simulink model "common_2"  (R2015b)
settings: Solver=ode4  StartTime=0.0  StopTime=10  FixedStep=0.005  RelTol=1e-3
undefined symbols (not defined in the file): dq_init, g, l1, l2, para, q_init
settings Model: Creator=Administrator  LastModifiedBy=Administrator

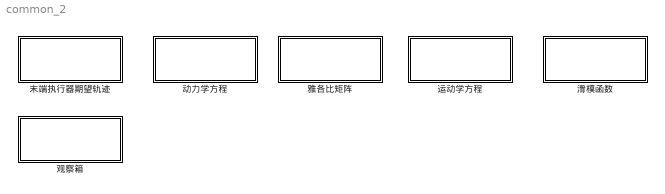
== system common_2 ==
  动力学方程 : Subsystem
      mask Display: disp('动力学方程')
  末端执行器期望轨迹 : Subsystem
      mask Display: disp('期望轨迹')
  滑模函数 : Subsystem
  观察箱 : Subsystem
  运动学方程 : Subsystem
      mask Display: disp('运动学方程')
  雅各比矩阵 : Subsystem
      mask Display: disp('雅各比矩阵')

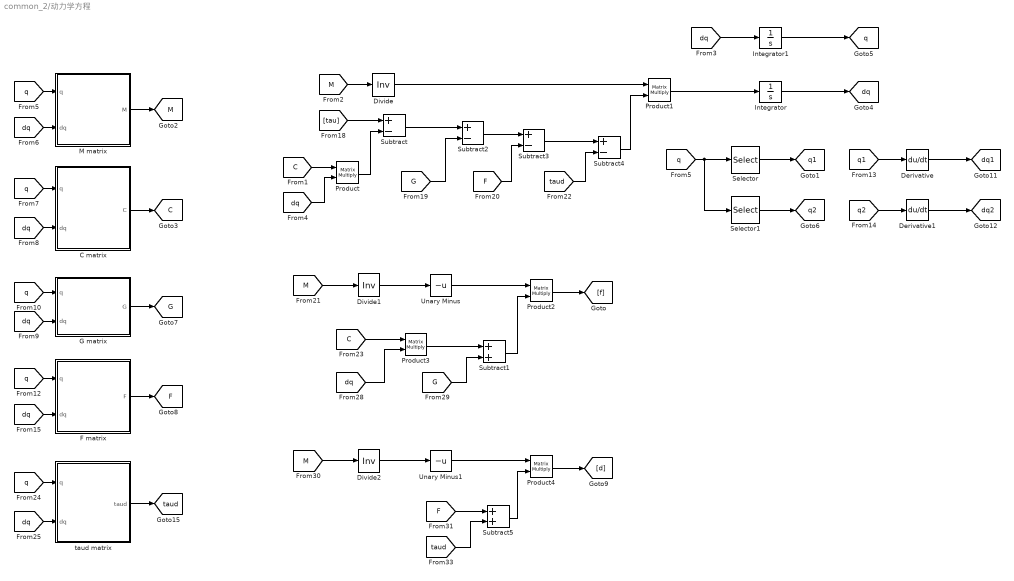
== system common_2/动力学方程 ==
  C matrix : Subsystem
  Derivative : Derivative
  Derivative1 : Derivative
  Divide : Product  Inputs=/  Multiplication=Matrix(*)
  Divide1 : Product  Inputs=/  Multiplication=Matrix(*)
  Divide2 : Product  Inputs=/  Multiplication=Matrix(*)
  F matrix : Subsystem
  G matrix : Subsystem
  Integrator : Integrator  InitialCondition=dq_init
  Integrator1 : Integrator  InitialCondition=q_init
  M matrix : Subsystem
  Product{,1..4} (5 alike) : Product  Multiplication=Matrix(*)
  Selector : Selector  InputPortWidth=2  IndexOptions=Index vector (dialog)  Indices=[1]  OutputSizes=1
  Selector1 : Selector  InputPortWidth=2  IndexOptions=Index vector (dialog)  Indices=[2]  OutputSizes=1
  Subtract{,2..4} (4 alike) : Sum  Inputs=+-
  Subtract1 : Sum
  Subtract5 : Sum
  Unary Minus : UnaryMinus
  Unary Minus1 : UnaryMinus
  taud matrix : Subsystem
  tag scope: C=global, F=global, G=global, M=global, dq1=global, dq2=global, dq=global, q1=global, q2=global, q=global, taud=global
  wires:
  Integrator/1 -> [dq]
  [dq] -> Integrator1/1
  Integrator1/1 -> [q]
  Selector/1 -> [q1]
  Selector1/1 -> [q2]
  [q] -> Selector1/1, Selector/1
  [q1] -> Derivative/1
  Derivative/1 -> [dq1]
  [q2] -> Derivative1/1
  Derivative1/1 -> [dq2]
  [q] -> C matrix/1(q)
  [dq] -> C matrix/2(dq)
  [q] -> M matrix/1(q)
  M matrix/1(M) -> [M]
  C matrix/1(C) -> [C]
  G matrix/1(G) -> [G]
  F matrix/1(F) -> [F]
  [M] -> Divide/1
  Product1/1 -> Integrator/1
  [q] -> G matrix/1(q)
  [q] -> F matrix/1(q)
  [dq] -> F matrix/2(dq)
  [q] -> taud matrix/1(q)
  [dq] -> taud matrix/2(dq)
  taud matrix/1(taud) -> [taud]
  Divide/1 -> Product1/1
  [tau] -> Subtract/1
  [C] -> Product/1
  [dq] -> Product/2
  Product/1 -> Subtract/2
  Subtract/1 -> Subtract2/1
  [G] -> Subtract2/2
  Subtract2/1 -> Subtract3/1
  [F] -> Subtract3/2
  Subtract3/1 -> Subtract4/1
  [taud] -> Subtract4/2
  Subtract4/1 -> Product1/2
  [dq] -> M matrix/2(dq)
  [dq] -> G matrix/2(dq)
  [M] -> Divide1/1
  Divide1/1 -> Unary Minus/1
  Unary Minus/1 -> Product2/1
  [C] -> Product3/1
  [dq] -> Product3/2
  Product3/1 -> Subtract1/1
  [G] -> Subtract1/2
  Subtract1/1 -> Product2/2
  Product2/1 -> [f]
  [M] -> Divide2/1
  Divide2/1 -> Unary Minus1/1
  Unary Minus1/1 -> Product4/1
  [F] -> Subtract5/1
  [taud] -> Subtract5/2
  Subtract5/1 -> Product4/2
  Product4/1 -> [d]

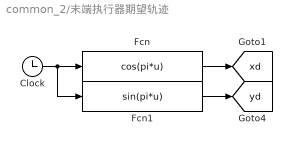
== system common_2/末端执行器期望轨迹 ==
  Clock : Clock
  Fcn : Fcn  Expr=cos(pi*u)
  Fcn1 : Fcn  Expr=sin(pi*u)
  tag scope: xd=global, yd=global
  wires:
  Clock/1 -> Fcn1/1, Fcn/1
  Fcn/1 -> [xd]
  Fcn1/1 -> [yd]

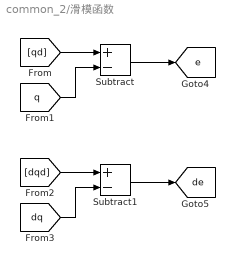
== system common_2/滑模函数 ==
  Subtract : Sum  Inputs=+-
  Subtract1 : Sum  Inputs=+-
  tag scope: de=global, e=global
  wires:
  [qd] -> Subtract/1
  [q] -> Subtract/2
  Subtract/1 -> [e]
  [dqd] -> Subtract1/1
  [dq] -> Subtract1/2
  Subtract1/1 -> [de]

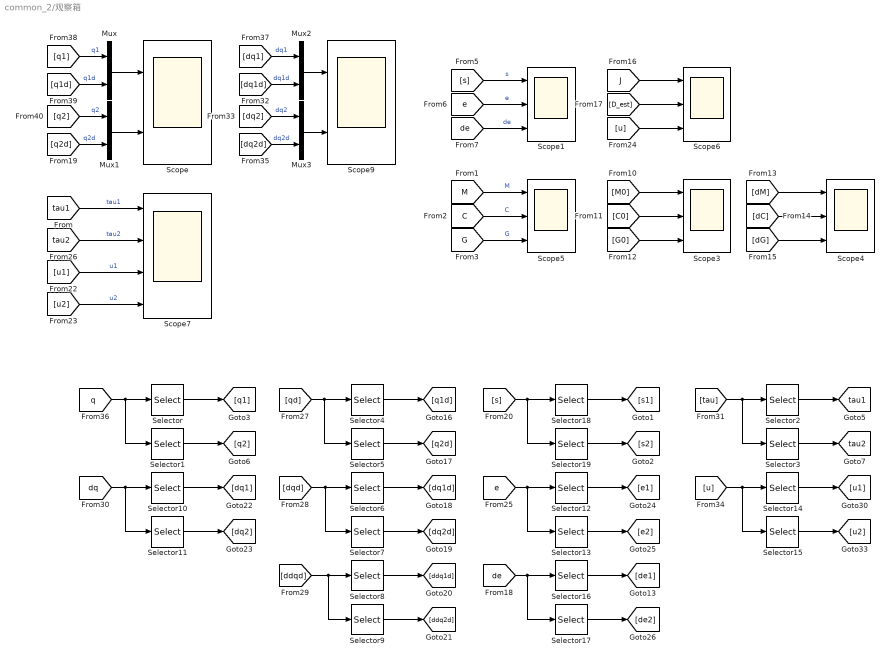
== system common_2/观察箱 ==
  Mux{,1..3} (4 alike) : Mux  Inputs=2
  Scope : Scope  NumInputPorts=2
  Scope{1,3..6} (5 alike) : Scope  NumInputPorts=3
  Scope7 : Scope  NumInputPorts=4
  Scope9 : Scope  NumInputPorts=2
  Selector{,2,4,6,8,10,12,14,16,18} (10 alike) : Selector  InputPortWidth=2  IndexOptions=Index vector (dialog)  Indices=[1]  OutputSizes=1
  Selector{1,3,5,7,9,11,13,15,17,19} (10 alike) : Selector  InputPortWidth=2  IndexOptions=Index vector (dialog)  Indices=[2]  OutputSizes=1
  tag scope: tau1=global, tau2=global
  wires:
  Selector/1 -> [q1]
  Selector1/1 -> [q2]
  [q1] -> Mux/1  "q1"
  [q1d] -> Mux/2  "q1d"
  Mux/1 -> Scope/1
  [q2] -> Mux1/1  "q2"
  [q2d] -> Mux1/2  "q2d"
  Mux1/1 -> Scope/2
  Selector4/1 -> [q1d]
  Selector5/1 -> [q2d]
  Selector6/1 -> [dq1d]
  Selector7/1 -> [dq2d]
  Selector8/1 -> [ddq1d]
  Selector9/1 -> [ddq2d]
  [qd] -> Selector5/1, Selector4/1
  [dqd] -> Selector7/1, Selector6/1
  [ddqd] -> Selector9/1, Selector8/1
  Selector10/1 -> [dq1]
  Selector11/1 -> [dq2]
  [q] -> Selector1/1, Selector/1
  [dq] -> Selector11/1, Selector10/1
  [dq1] -> Mux2/1  "dq1"
  [dq1d] -> Mux2/2  "dq1d"
  Mux2/1 -> Scope9/1
  [dq2] -> Mux3/1  "dq2"
  [dq2d] -> Mux3/2  "dq2d"
  Mux3/1 -> Scope9/2
  Selector13/1 -> [e2]
  [e] -> Selector13/1, Selector12/1
  Selector12/1 -> [e1]
  Selector17/1 -> [de2]
  [de] -> Selector16/1, Selector17/1
  Selector16/1 -> [de1]
  Selector2/1 -> [tau1]
  Selector3/1 -> [tau2]
  [tau] -> Selector3/1, Selector2/1
  Selector14/1 -> [u1]
  Selector15/1 -> [u2]
  [u] -> Selector14/1, Selector15/1
  [tau1] -> Scope7/1  "tau1"
  [tau2] -> Scope7/2  "tau2"
  [u1] -> Scope7/3  "u1"
  [u2] -> Scope7/4  "u2"
  [M] -> Scope5/1  "M"
  [C] -> Scope5/2  "C"
  [G] -> Scope5/3  "G"
  [s] -> Scope1/1  "s"
  [e] -> Scope1/2  "e"
  [de] -> Scope1/3  "de"
  [M0] -> Scope3/1
  [C0] -> Scope3/2
  [G0] -> Scope3/3
  [dM] -> Scope4/1
  [dC] -> Scope4/2
  [dG] -> Scope4/3
  [J] -> Scope6/1
  [D_est] -> Scope6/2
  [u] -> Scope6/3
  Selector19/1 -> [s2]
  [s] -> Selector18/1, Selector19/1
  Selector18/1 -> [s1]

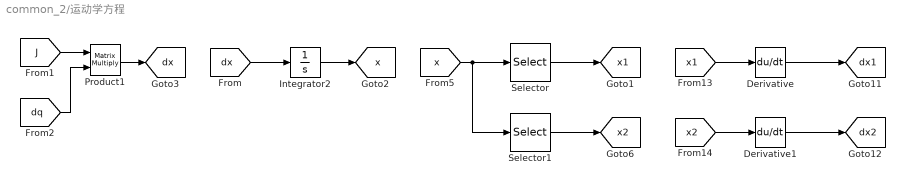
== system common_2/运动学方程 ==
  Derivative : Derivative
  Derivative1 : Derivative
  Integrator2 : Integrator  InitialCondition=dq_init
  Product1 : Product  Multiplication=Matrix(*)
  Selector : Selector  InputPortWidth=2  IndexOptions=Index vector (dialog)  Indices=[1]  OutputSizes=1
  Selector1 : Selector  InputPortWidth=2  IndexOptions=Index vector (dialog)  Indices=[2]  OutputSizes=1
  tag scope: dx1=global, dx2=global, dx=global, x1=global, x2=global, x=global
  wires:
  Derivative1/1 -> [dx2]
  [x2] -> Derivative1/1
  Derivative/1 -> [dx1]
  [x1] -> Derivative/1
  [x] -> Selector/1, Selector1/1
  Selector1/1 -> [x2]
  Selector/1 -> [x1]
  Integrator2/1 -> [x]
  [J] -> Product1/1
  [dq] -> Product1/2
  Product1/1 -> [dx]
  [dx] -> Integrator2/1

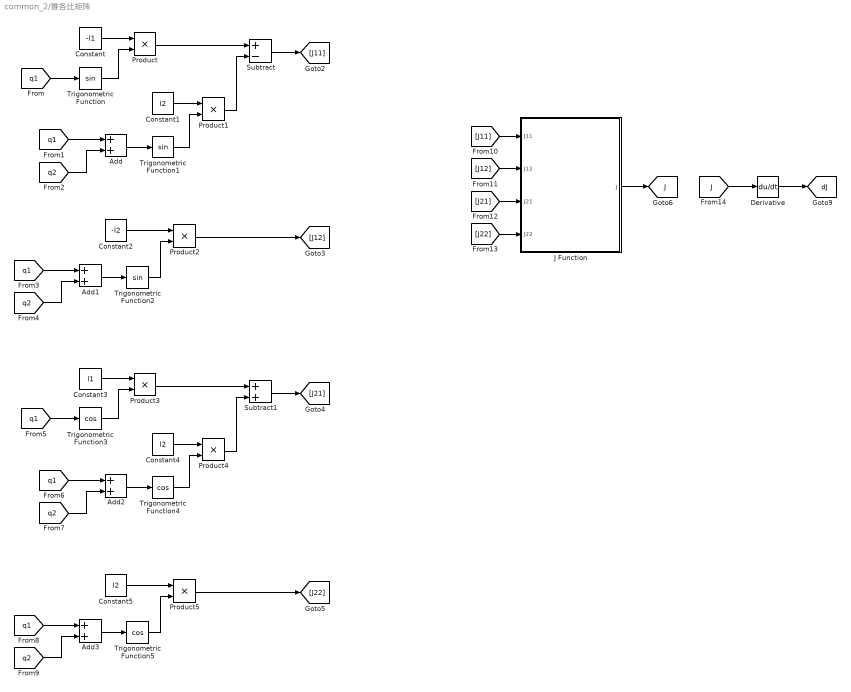
== system common_2/雅各比矩阵 ==
  Add{,1..3} (4 alike) : Sum
  Constant : Constant  Value=-l1
  Constant1 : Constant  Value=l2
  Constant2 : Constant  Value=-l2
  Constant3 : Constant  Value=l1
  Constant4 : Constant  Value=l2
  Constant5 : Constant  Value=l2
  Derivative : Derivative
  J Function : MATLAB Function  TreatAsAtomicUnit=on
  Product{,1..5} (6 alike) : Product
  Subtract : Sum  Inputs=+-
  Subtract1 : Sum
  Trigonometric Function : Trigonometry
  Trigonometric Function1 : Trigonometry
  Trigonometric Function2 : Trigonometry
  Trigonometric Function3 : Trigonometry  Operator=cos
  Trigonometric Function4 : Trigonometry  Operator=cos
  Trigonometric Function5 : Trigonometry  Operator=cos
  tag scope: J=global, dJ=global
  wires:
  Constant/1 -> Product/1
  Trigonometric Function/1 -> Product/2
  [q1] -> Trigonometric Function/1
  Product/1 -> Subtract/1
  Constant1/1 -> Product1/1
  Trigonometric Function1/1 -> Product1/2
  Product1/1 -> Subtract/2
  Add/1 -> Trigonometric Function1/1
  [q1] -> Add/1
  [q2] -> Add/2
  Subtract/1 -> [J11]
  Constant2/1 -> Product2/1
  Add1/1 -> Trigonometric Function2/1
  [q1] -> Add1/1
  [q2] -> Add1/2
  Trigonometric Function2/1 -> Product2/2
  Product2/1 -> [J12]
  Constant3/1 -> Product3/1
  Trigonometric Function3/1 -> Product3/2
  [q1] -> Trigonometric Function3/1
  Product3/1 -> Subtract1/1
  Constant4/1 -> Product4/1
  Trigonometric Function4/1 -> Product4/2
  Product4/1 -> Subtract1/2
  Add2/1 -> Trigonometric Function4/1
  [q1] -> Add2/1
  [q2] -> Add2/2
  Subtract1/1 -> [J21]
  Constant5/1 -> Product5/1
  Add3/1 -> Trigonometric Function5/1
  [q1] -> Add3/1
  [q2] -> Add3/2
  Trigonometric Function5/1 -> Product5/2
  Product5/1 -> [J22]
  [J11] -> J Function/1(J11)
  [J12] -> J Function/2(J12)
  [J21] -> J Function/3(J21)
  [J22] -> J Function/4(J22)
  J Function/1(J) -> [J]
  [J] -> Derivative/1
  Derivative/1 -> [dJ]

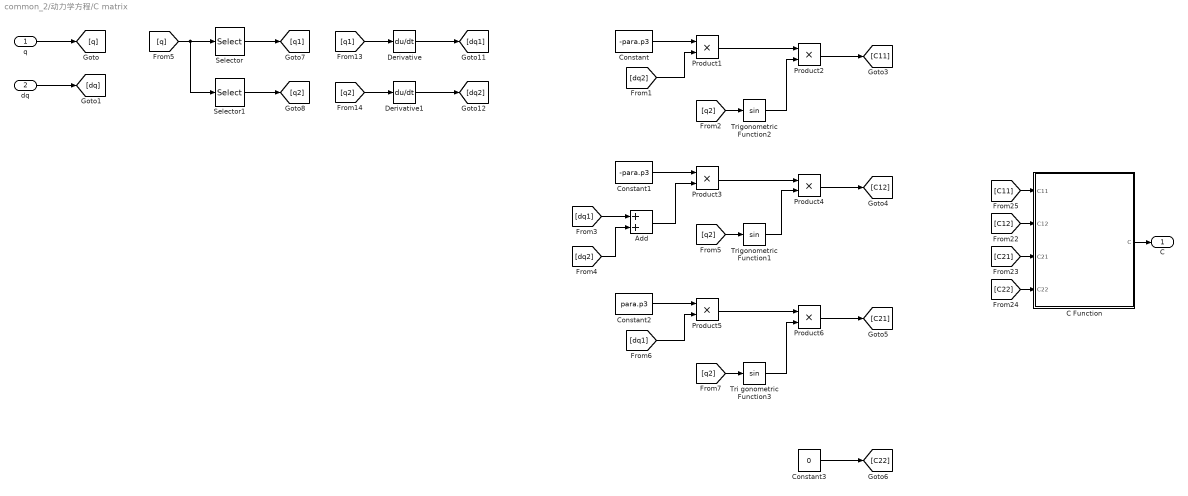
== system common_2/动力学方程/C matrix ==
  q : Inport
  dq : Inport  Port=2
  Add : Sum
  C Function : MATLAB Function  TreatAsAtomicUnit=on
  Constant : Constant  Value=-para.p3
  Constant1 : Constant  Value=-para.p3
  Constant2 : Constant  Value=para.p3
  Constant3 : Constant  Value=0
  Derivative : Derivative
  Derivative1 : Derivative
  Product{1..6} (6 alike) : Product
  Selector : Selector  InputPortWidth=2  IndexOptions=Index vector (dialog)  Indices=[1]  OutputSizes=1
  Selector1 : Selector  InputPortWidth=2  IndexOptions=Index vector (dialog)  Indices=[2]  OutputSizes=1
  Tri gonometric Function3 : Trigonometry
  Trigonometric Function1 : Trigonometry
  Trigonometric Function2 : Trigonometry
  C : Outport
  wires:
  [C11] -> C Function/1(C11)
  [C12] -> C Function/2(C12)
  [C21] -> C Function/3(C21)
  [C22] -> C Function/4(C22)
  C Function/1(C) -> C/1
  q/1 -> [q]
  dq/1 -> [dq]
  Constant/1 -> Product1/1
  [dq2] -> Product1/2
  Product1/1 -> Product2/1
  [q2] -> Trigonometric Function2/1
  Trigonometric Function2/1 -> Product2/2
  Selector/1 -> [q1]
  Selector1/1 -> [q2]
  [q] -> Selector1/1, Selector/1
  [q1] -> Derivative/1
  Derivative/1 -> [dq1]
  [q2] -> Derivative1/1
  Derivative1/1 -> [dq2]
  Product2/1 -> [C11]
  Constant1/1 -> Product3/1
  [dq1] -> Add/1
  [dq2] -> Add/2
  Add/1 -> Product3/2
  Product3/1 -> Product4/1
  [q2] -> Trigonometric Function1/1
  Trigonometric Function1/1 -> Product4/2
  Product4/1 -> [C12]
  Constant2/1 -> Product5/1
  [dq1] -> Product5/2
  Product5/1 -> Product6/1
  [q2] -> Tri gonometric Function3/1
  Tri gonometric Function3/1 -> Product6/2
  Product6/1 -> [C21]
  Constant3/1 -> [C22]

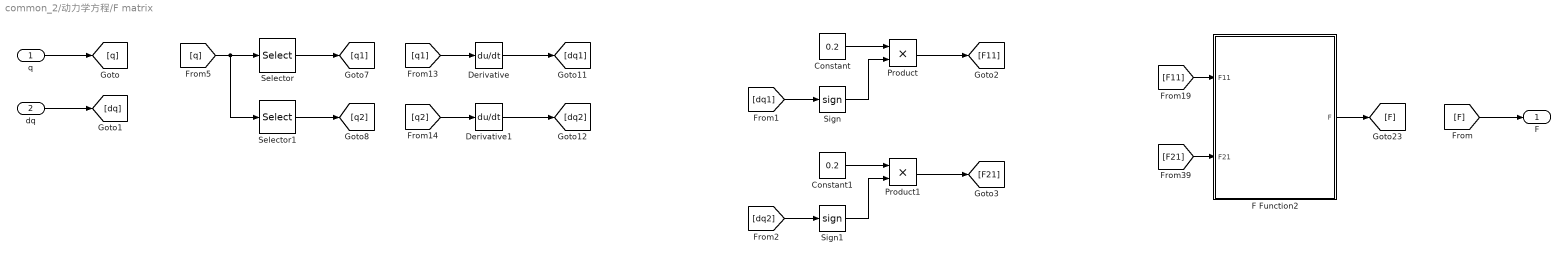
== system common_2/动力学方程/F matrix ==
  q : Inport
  dq : Inport  Port=2
  Constant : Constant  Value=0.2
  Constant1 : Constant  Value=0.2
  Derivative : Derivative
  Derivative1 : Derivative
  F Function2 : MATLAB Function  TreatAsAtomicUnit=on
  Product : Product
  Product1 : Product
  Selector : Selector  InputPortWidth=2  IndexOptions=Index vector (dialog)  Indices=[1]  OutputSizes=1
  Selector1 : Selector  InputPortWidth=2  IndexOptions=Index vector (dialog)  Indices=[2]  OutputSizes=1
  Sign : Signum
  Sign1 : Signum
  F : Outport
  wires:
  [F] -> F/1
  F Function2/1(F) -> [F]
  [F11] -> F Function2/1(F11)
  [F21] -> F Function2/2(F21)
  q/1 -> [q]
  dq/1 -> [dq]
  Selector/1 -> [q1]
  Selector1/1 -> [q2]
  [q] -> Selector1/1, Selector/1
  [q1] -> Derivative/1
  Derivative/1 -> [dq1]
  [q2] -> Derivative1/1
  Derivative1/1 -> [dq2]
  Constant/1 -> Product/1
  Sign/1 -> Product/2
  [dq1] -> Sign/1
  Product/1 -> [F11]
  Constant1/1 -> Product1/1
  Sign1/1 -> Product1/2
  [dq2] -> Sign1/1
  Product1/1 -> [F21]

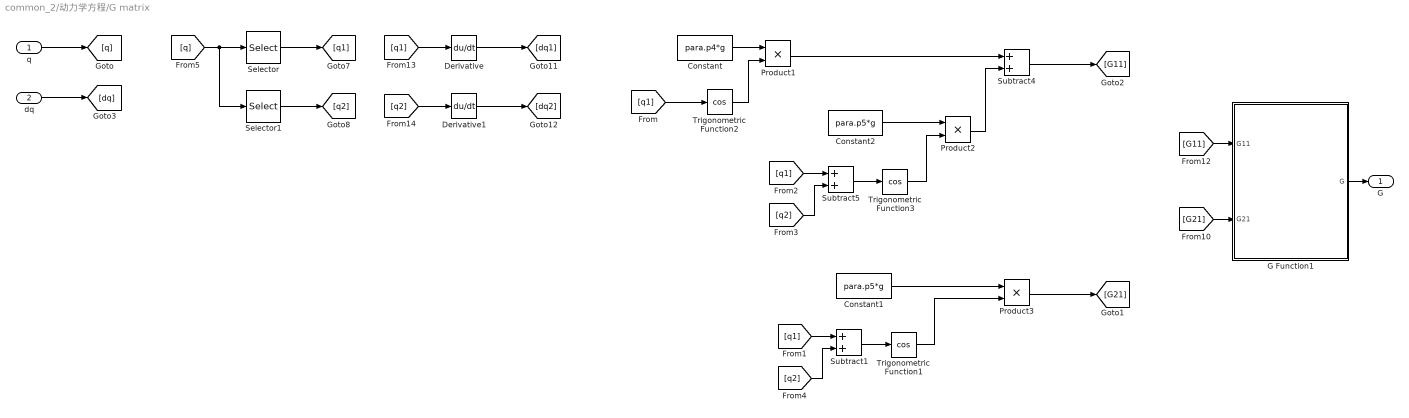
== system common_2/动力学方程/G matrix ==
  q : Inport
  dq : Inport  Port=2
  Constant : Constant  Value=para.p4*g
  Constant1 : Constant  Value=para.p5*g
  Constant2 : Constant  Value=para.p5*g
  Derivative : Derivative
  Derivative1 : Derivative
  G Function1 : MATLAB Function  TreatAsAtomicUnit=on
  Product1 : Product
  Product2 : Product
  Product3 : Product
  Selector : Selector  InputPortWidth=2  IndexOptions=Index vector (dialog)  Indices=[1]  OutputSizes=1
  Selector1 : Selector  InputPortWidth=2  IndexOptions=Index vector (dialog)  Indices=[2]  OutputSizes=1
  Subtract1 : Sum
  Subtract4 : Sum
  Subtract5 : Sum
  Trigonometric Function1 : Trigonometry  Operator=cos
  Trigonometric Function2 : Trigonometry  Operator=cos
  Trigonometric Function3 : Trigonometry  Operator=cos
  G : Outport
  wires:
  [G11] -> G Function1/1(G11)
  [G21] -> G Function1/2(G21)
  G Function1/1(G) -> G/1
  Constant/1 -> Product1/1
  Trigonometric Function2/1 -> Product1/2
  [q1] -> Trigonometric Function2/1
  Product1/1 -> Subtract4/1
  Constant2/1 -> Product2/1
  Subtract5/1 -> Trigonometric Function3/1
  [q1] -> Subtract5/1
  [q2] -> Subtract5/2
  Trigonometric Function3/1 -> Product2/2
  Product2/1 -> Subtract4/2
  Subtract4/1 -> [G11]
  Constant1/1 -> Product3/1
  Subtract1/1 -> Trigonometric Function1/1
  [q1] -> Subtract1/1
  [q2] -> Subtract1/2
  Trigonometric Function1/1 -> Product3/2
  Product3/1 -> [G21]
  q/1 -> [q]
  dq/1 -> [dq]
  Selector/1 -> [q1]
  Selector1/1 -> [q2]
  [q] -> Selector1/1, Selector/1
  [q1] -> Derivative/1
  Derivative/1 -> [dq1]
  [q2] -> Derivative1/1
  Derivative1/1 -> [dq2]

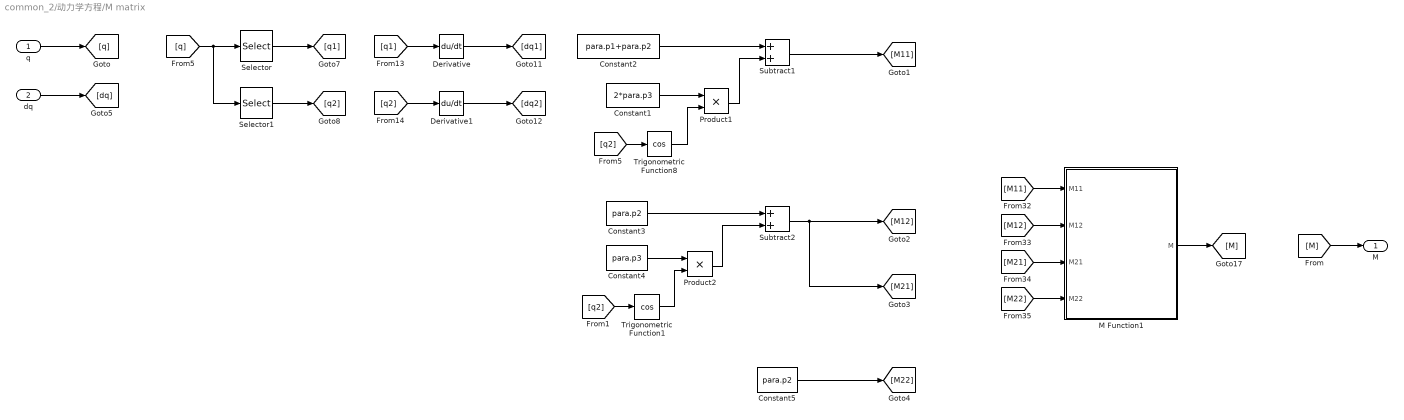
== system common_2/动力学方程/M matrix ==
  q : Inport
  dq : Inport  Port=2
  Constant1 : Constant  Value=2*para.p3
  Constant2 : Constant  Value=para.p1+para.p2
  Constant3 : Constant  Value=para.p2
  Constant4 : Constant  Value=para.p3
  Constant5 : Constant  Value=para.p2
  Derivative : Derivative
  Derivative1 : Derivative
  M Function1 : MATLAB Function  TreatAsAtomicUnit=on
  Product1 : Product
  Product2 : Product
  Selector : Selector  InputPortWidth=2  IndexOptions=Index vector (dialog)  Indices=[1]  OutputSizes=1
  Selector1 : Selector  InputPortWidth=2  IndexOptions=Index vector (dialog)  Indices=[2]  OutputSizes=1
  Subtract1 : Sum
  Subtract2 : Sum
  Trigonometric Function1 : Trigonometry  Operator=cos
  Trigonometric Function8 : Trigonometry  Operator=cos
  M : Outport
  wires:
  M Function1/1(M) -> [M]
  [M11] -> M Function1/1(M11)
  [M12] -> M Function1/2(M12)
  [M21] -> M Function1/3(M21)
  [M22] -> M Function1/4(M22)
  [q2] -> Trigonometric Function8/1
  [M] -> M/1
  Constant2/1 -> Subtract1/1
  Constant1/1 -> Product1/1
  Trigonometric Function8/1 -> Product1/2
  Product1/1 -> Subtract1/2
  Subtract2/1 -> [M21], [M12]
  Constant5/1 -> [M22]
  Subtract1/1 -> [M11]
  Constant3/1 -> Subtract2/1
  Constant4/1 -> Product2/1
  [q2] -> Trigonometric Function1/1
  Trigonometric Function1/1 -> Product2/2
  Product2/1 -> Subtract2/2
  q/1 -> [q]
  dq/1 -> [dq]
  Selector/1 -> [q1]
  Selector1/1 -> [q2]
  [q] -> Selector1/1, Selector/1
  [q1] -> Derivative/1
  Derivative/1 -> [dq1]
  [q2] -> Derivative1/1
  Derivative1/1 -> [dq2]

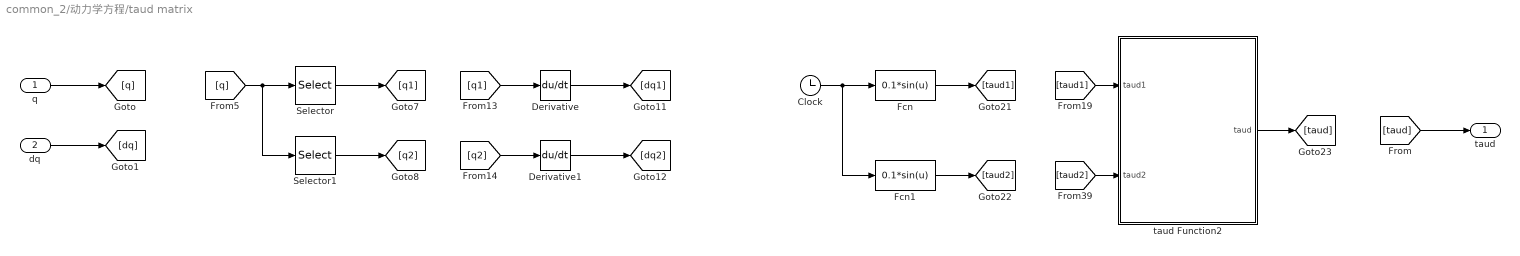
== system common_2/动力学方程/taud matrix ==
  q : Inport
  dq : Inport  Port=2
  Clock : Clock
  Derivative : Derivative
  Derivative1 : Derivative
  Fcn : Fcn  Expr=0.1*sin(u)
  Fcn1 : Fcn  Expr=0.1*sin(u)
  Selector : Selector  InputPortWidth=2  IndexOptions=Index vector (dialog)  Indices=[1]  OutputSizes=1
  Selector1 : Selector  InputPortWidth=2  IndexOptions=Index vector (dialog)  Indices=[2]  OutputSizes=1
  taud Function2 : MATLAB Function  TreatAsAtomicUnit=on
  taud : Outport
  wires:
  [taud2] -> taud Function2/2(taud2)
  [taud1] -> taud Function2/1(taud1)
  taud Function2/1(taud) -> [taud]
  [taud] -> taud/1
  q/1 -> [q]
  dq/1 -> [dq]
  Selector/1 -> [q1]
  Selector1/1 -> [q2]
  [q] -> Selector1/1, Selector/1
  [q1] -> Derivative/1
  Derivative/1 -> [dq1]
  [q2] -> Derivative1/1
  Derivative1/1 -> [dq2]
  Clock/1 -> Fcn1/1, Fcn/1
  Fcn/1 -> [taud1]
  Fcn1/1 -> [taud2]

== matlab function common_2/雅各比矩阵/J Function ==
  data: J11 input; J output; J12 input; J21 input; J22 input
function J = fcn(J11,J12,J21,J22)
%#codegen

J = [J11 J12;J21 J22];

== matlab function common_2/动力学方程/G matrix/G Function1 ==
  data: G11 input; G output; G21 input
function G = fcn(G11,G21)
%#codegen

G = [G11;G21];

== matlab function common_2/动力学方程/C matrix/C Function ==
  data: C11 input; C output; C12 input; C21 input; C22 input
function C = fcn(C11,C12,C21,C22)
%#codegen

C = [C11 C12;C21 C22];

== matlab function common_2/动力学方程/M matrix/M Function1 ==
  data: M11 input; M output; M12 input; M21 input; M22 input
function M = fcn(M11,M12,M21,M22)
%#codegen

M = [M11 M12;M21 M22];

== matlab function common_2/动力学方程/F matrix/F Function2 ==
  data: F11 input; F output; F21 input
function F = fcn(F11,F21)
%#codegen

F = [F11;F21];

== matlab function common_2/动力学方程/taud matrix/taud Function2 ==
  data: taud1 input; taud output; taud2 input
function taud = fcn(taud1,taud2)
%#codegen

taud = [taud1;taud2];
